simulink subsystem "AGV_Dynamic_Simulation"  (R2024b)
settings: Solver=VariableStepAuto  StartTime=0.0  StopTime=10.0  RelTol=1e-3
model mask{Ts=0.5, InitialSpeed=[0 0], InitialPose=[0 0 0]}
  mask prompts: Ts "Sample Time (s)"; InitialSpeed "Initial Speed (m/s, rad/s)"; InitialPose "Initial Pose (m,m,rad)"
settings Model: Creator=marti  LastModifiedBy=marti

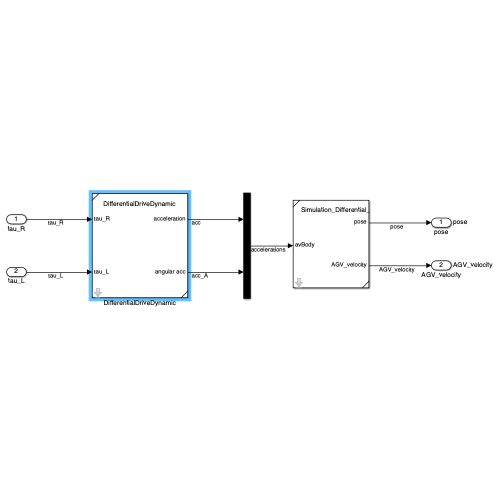
[thumbnail: Simulink's stored preview of the top-level diagram]
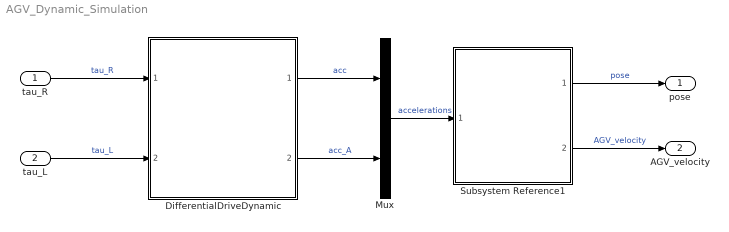
== system AGV_Dynamic_Simulation ==
  tau_R : Inport  PortDimensions=1  SampleTime=Ts
  tau_L : Inport  Port=2  PortDimensions=1  SampleTime=Ts
  DifferentialDriveDynamic : Subsystem  ReferencedSubsystem=DifferentialDriveDynamic  L=0.81  J=17.67  M=115  R=0.26/2  max_speed=[-Inf Inf]  max_accel=[-Inf Inf]
  Mux : Mux  Inputs=2
  Subsystem Reference1 : Subsystem  ReferencedSubsystem=Simulation_Differential_AGV  poseInit=InitialPose  vInit=InitialSpeed  Ts=Ts  speedLimits=[-inf inf]
  pose : Outport  SignalName=pose  PortDimensions=3  SampleTime=Ts
  AGV_velocity : Outport  Port=2  SignalName=AGV_velocity  SampleTime=Ts
  wires:
  DifferentialDriveDynamic/2 -> Mux/2  "acc_A"
  Subsystem Reference1/2 -> AGV_velocity/1  "AGV_velocity"
  tau_L/1 -> DifferentialDriveDynamic/2  "tau_L"
  tau_R/1 -> DifferentialDriveDynamic/1  "tau_R"
  DifferentialDriveDynamic/1 -> Mux/1  "acc"
  Subsystem Reference1/1 -> pose/1  "pose"
  Mux/1 -> Subsystem Reference1/1  "accelerations"
